simulink model "scon2_L8_1ponto4_simulink"  (R2024a)
settings: Solver=ode4  StartTime=0.0  StopTime=10.0  FixedStep=0.001  RelTol=1e-3
values from neighbouring files (symbols this model uses):
  A = [-9, 1, 0; -26, 0, 1; -24, 0, 0]    [scon_L8_1ponto4.m]
  B = [0; 0; 2]    [scon_L8_1ponto4.m]
  Kc = K(1:3)    [scon_L8_1ponto4.m]
  Ki = -K(4)    [scon_L8_1ponto4.m]
settings Model: Creator=NIA  LastModifiedBy=Carlos Augusto
settings ModelReferenceCC: EnableRefExpFcnMdlSchedulingChecks=on
settings RTWCC: GPUComputeCapability=3.5

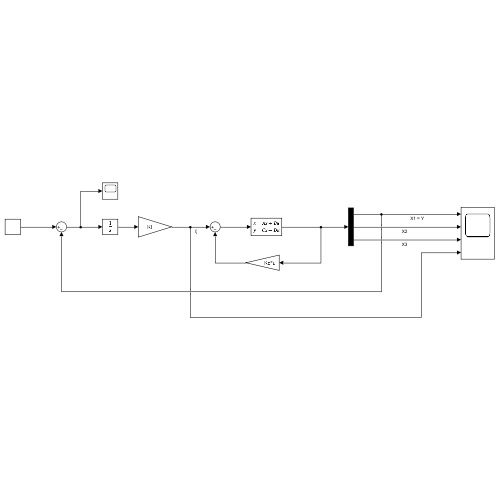
[thumbnail: Simulink's stored preview of the top-level diagram]
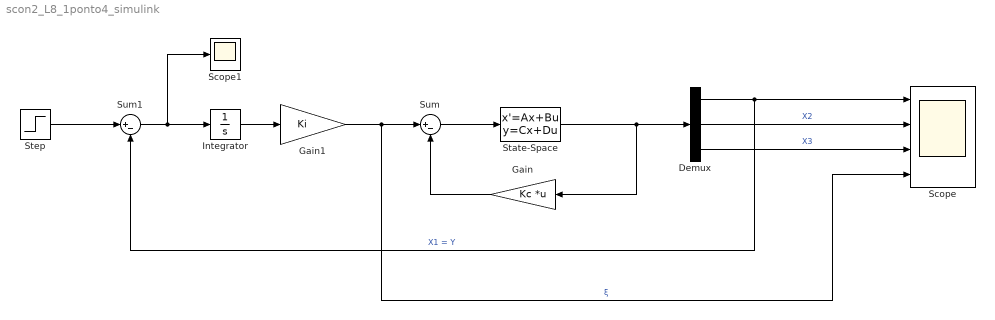
== system scon2_L8_1ponto4_simulink ==
  Demux : Demux  Outputs=3
  Gain : Gain  Gain=Kc  Multiplication=Matrix(K*u)
  Gain1 : Gain  Gain=Ki
  Integrator : Integrator
  Scope : Scope  NumInputPorts=4
  Scope1 : Scope
  State-Space : StateSpace  A=A  B=B  C=eye(3)  D=zeros(3,1)  InitialCondition=0
  Step : Step  SampleTime=0
  Sum : Sum  Inputs=|+-
  Sum1 : Sum  Inputs=|+-
  wires:
  State-Space/1 -> Gain/1, Demux/1
  Demux/2 -> Scope/2  "X2"
  Demux/1 -> Scope/1, Sum1/2  "X1 = Y"
  Demux/3 -> Scope/3  "X3"
  Gain/1 -> Sum/2
  Sum/1 -> State-Space/1
  Gain1/1 -> Scope/4, Sum/1  "ξ"
  Integrator/1 -> Gain1/1
  Step/1 -> Sum1/1
  Sum1/1 -> Scope1/1, Integrator/1
